simulink model "lab3_close_loop_pwm"  (R2023a)
settings: Solver=VariableStepAuto  StartTime=0.0  StopTime=10.0  RelTol=1e-3
model workspace (MAT data in the model file):
  E = 0.05
values from neighbouring files (symbols this model uses):
  anum = 0.3    [lab3.m]
  den = [1 0 w0^2]    [lab3.m]
  denD = cell2mat(denD)    [lab3.m]
  num = G*w0^2    (= 4)    [lab3.m]
  numD = cell2mat(numD)    [lab3.m]
  Ts = 0.1    [lab3.m]
libraries: simulink x1
settings Model: Creator=dgkegkas2023  LastModifiedBy=dgkegkas2023

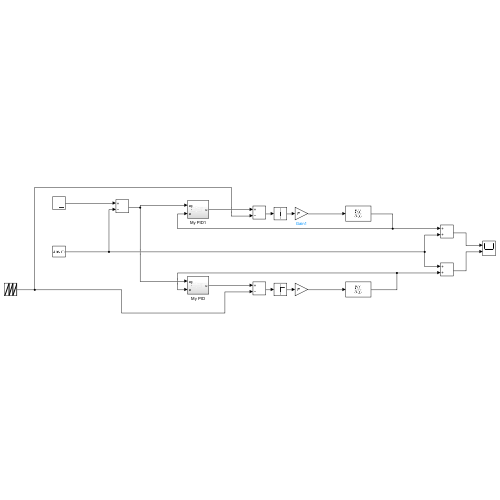
[thumbnail: Simulink's stored preview of the top-level diagram]
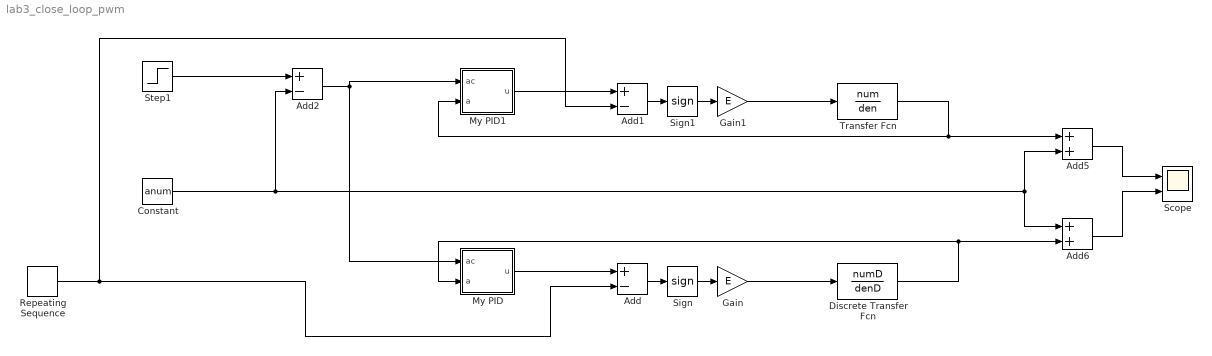
== system lab3_close_loop_pwm ==
  Add : Sum  Inputs=+-
  Add1 : Sum  Inputs=+-
  Add2 : Sum  Inputs=+-
  Add5 : Sum
  Add6 : Sum
  Constant : Constant  Value=anum
  Discrete Transfer Fcn : DiscreteTransferFcn  Numerator=numD  Denominator=denD
  Gain : Gain  Gain=E
  Gain1 : Gain  Gain=E
  My PID : Subsystem
  My PID1 : Subsystem
  Repeating Sequence : simulink/Sources/Repeating Sequence  rep_seq_t=[0 0.02]  rep_seq_y=[-E E]
  Scope : Scope  NumInputPorts=2
  Sign : Signum
  Sign1 : Signum
  Step1 : Step  Before=0.3  After=0.27  SampleTime=Ts
  Transfer Fcn : TransferFcn  Numerator=num  Denominator=den
  wires:
  Constant/1 -> Add2/2, Add6/1, Add5/2
  Discrete Transfer Fcn/1 -> My PID/2(a), Add6/2
  Add6/1 -> Scope/2
  Add5/1 -> Scope/1
  Step1/1 -> Add2/1
  Add2/1 -> My PID/1(ac), My PID1/1(ac)
  Transfer Fcn/1 -> My PID1/2(a), Add5/1
  My PID/1(u) -> Add/1
  Repeating Sequence/1 -> Add1/2, Add/2
  Add/1 -> Sign/1
  Sign/1 -> Gain/1
  Gain/1 -> Discrete Transfer Fcn/1
  Add1/1 -> Sign1/1
  Sign1/1 -> Gain1/1
  My PID1/1(u) -> Add1/1
  Gain1/1 -> Transfer Fcn/1

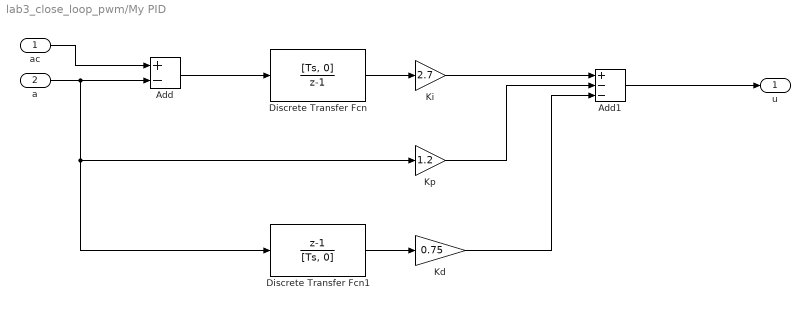
== system lab3_close_loop_pwm/My PID ==
  ac : Inport
  a : Inport  Port=2
  Add : Sum  Inputs=+-
  Add1 : Sum  Inputs=+--
  Discrete Transfer Fcn : DiscreteTransferFcn  Numerator=[Ts, 0]  Denominator=[1, -1]  SampleTime=Ts
  Discrete Transfer Fcn1 : DiscreteTransferFcn  Numerator=[1, -1]  Denominator=[Ts, 0]  SampleTime=Ts
  Kd : Gain  Gain=0.75
  Ki : Gain  Gain=2.7
  Kp : Gain  Gain=1.2
  u : Outport
  wires:
  ac/1 -> Add/1
  a/1 -> Kp/1, Discrete Transfer Fcn1/1, Add/2
  Discrete Transfer Fcn/1 -> Ki/1
  Discrete Transfer Fcn1/1 -> Kd/1
  Kp/1 -> Add1/2
  Add1/1 -> u/1
  Ki/1 -> Add1/1
  Kd/1 -> Add1/3
  Add/1 -> Discrete Transfer Fcn/1

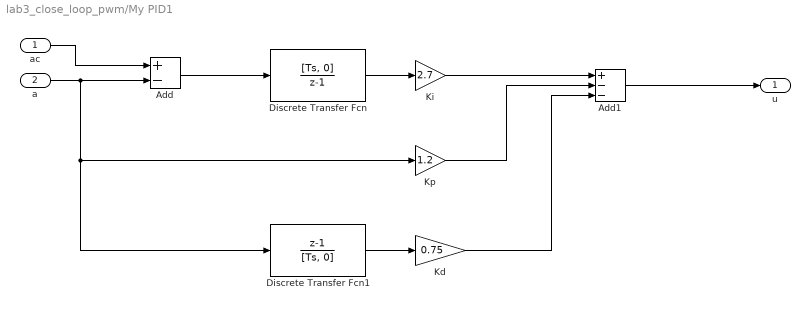
== system lab3_close_loop_pwm/My PID1 ==
  ac : Inport
  a : Inport  Port=2
  Add : Sum  Inputs=+-
  Add1 : Sum  Inputs=+--
  Discrete Transfer Fcn : DiscreteTransferFcn  Numerator=[Ts, 0]  Denominator=[1, -1]  SampleTime=Ts
  Discrete Transfer Fcn1 : DiscreteTransferFcn  Numerator=[1, -1]  Denominator=[Ts, 0]  SampleTime=Ts
  Kd : Gain  Gain=0.75
  Ki : Gain  Gain=2.7
  Kp : Gain  Gain=1.2
  u : Outport
  wires:
  ac/1 -> Add/1
  a/1 -> Kp/1, Discrete Transfer Fcn1/1, Add/2
  Discrete Transfer Fcn/1 -> Ki/1
  Discrete Transfer Fcn1/1 -> Kd/1
  Kp/1 -> Add1/2
  Add1/1 -> u/1
  Ki/1 -> Add1/1
  Kd/1 -> Add1/3
  Add/1 -> Discrete Transfer Fcn/1
